simulink model "NLPID"  (Simulink 7.3)
settings: Solver=ode5  StartTime=0.0  StopTime=inf  FixedStep=0.1  RelTol=1e-3
undefined symbols (not defined in the file): eta1_0_real, v1_0_real, velocitySatValues1
libraries: simulink x35, dspmtrx3 x15, simulink_extras x13, dspindex x5, marine_gnc x4, dspinverses x2
(part 4 of 4)

== system NLPID/Control Systems/Nonlinear PID/Thruster allocation/f_act to u_act/f_4 to u_4 ==
  note: If < 0: control input is 1
      | if = 0 control input is 2
      | if > 0: control input is 3
  note: Check if the input value is less, equal or greater then zero
  note: The mapping is divided into 3 parts:
      | Negative, zero and positive
  f_4 : Inport
  Dead Zone : DeadZone  LowerValue=-0.001  UpperValue=0.001  SaturateOnIntegerOverflow=on
  Gain : Gain  Gain=2  ParameterDataType=fixdt(1, 16)  ParameterScaling=2^0  OutDataType=fixdt(1, 16)  OutScaling=2^0
  Gain1 : Gain  Gain=3  ParameterDataType=fixdt(1, 16)  ParameterScaling=2^0  OutDataType=fixdt(1, 16)  OutScaling=2^0
  If < 0 : simulink/Logic and Bit Operations/Compare To Constant  SystemSampleTime=-1  relop=<  const=0  LogicOutDataTypeMode=uint8
  If > 0 : simulink/Logic and Bit Operations/Compare To Constant  SystemSampleTime=-1  relop=>  const=0  LogicOutDataTypeMode=uint8
  Multiport Switch : MultiPortSwitch  OutDataType=fixdt(1, 16)  OutScaling=2^0
  Sum : Sum  Inputs=+++  OutDataType=fixdt(1, 16)  OutScaling=2^0
  f_4 < 0 : Lookup  InputValues=|  Table=|  LookUpMeth=Interpolation-Use End Values  OutDataType=fixdt(1, 16)  OutScaling=2^0
      InputValues=|
      | [-1.249
      | -1.225
      | -1.094
      | -0.896
      | -0.696
      | -0.502
      | -0.314
      | -0.169
      | -0.042
      | 0.000]
      Table=|
      | [-0.9000
      |    -0.8000
      |    -0.7000
      |    -0.6000
      |    -0.5000
      |    -0.4000
      |    -0.3000
      |    -0.2000
      |    -0.1000
      |    -0.0674]
  f_4 = 0 : Constant  Value=0  OutDataType=fixdt(1, 16)  OutScaling=2^0
  f_4 > 0 : Lookup  InputValues=|  Table=|  LookUpMeth=Interpolation-Use End Values  OutDataType=fixdt(1, 16)  OutScaling=2^0
      InputValues=|
      | [0.000
      | 0.063
      | 0.107
      | 0.274
      | 0.441
      | 0.599
      | 0.731]
      Table=|
      | [0.3588
      |     0.5000
      |     0.6000
      |     0.7000
      |     0.8000
      |     0.9000
      |     1.0000]
  if == 0 : simulink/Logic and Bit Operations/Compare To Zero  SystemSampleTime=-1  relop===  LogicOutDataTypeMode=uint8
  u_4 : Outport
  wires:
  f_4 > 0/1 -> Multiport Switch/4
  f_4 = 0/1 -> Multiport Switch/3
  f_4 < 0/1 -> Multiport Switch/2
  f_4/1 -> f_4 > 0/1, f_4 < 0/1, Dead Zone/1
  If < 0/1 -> Sum/1
  if == 0/1 -> Gain/1
  If > 0/1 -> Gain1/1
  Sum/1 -> Multiport Switch/1
  Gain/1 -> Sum/2
  Gain1/1 -> Sum/3
  Multiport Switch/1 -> u_4/1
  Dead Zone/1 -> If > 0/1, if == 0/1, If < 0/1

== system NLPID/Control Systems/Nonlinear PID/Thruster allocation/f_act to u_act/f_5 to u_5 ==
  note: The mapping is divided into 3 parts:
      | Negative, zero and positive
  note: Check if the input value is less, equal or greater then zero
  note: If < 0: control input is 1
      | if = 0 control input is 2
      | if > 0: control input is 3
  f_5 : Inport
  Dead Zone : DeadZone  LowerValue=-0.001  UpperValue=0.001  SaturateOnIntegerOverflow=on
  Gain : Gain  Gain=2  ParameterDataType=fixdt(1, 16)  ParameterScaling=2^0  OutDataType=fixdt(1, 16)  OutScaling=2^0
  Gain1 : Gain  Gain=3  ParameterDataType=fixdt(1, 16)  ParameterScaling=2^0  OutDataType=fixdt(1, 16)  OutScaling=2^0
  If < 0 : simulink/Logic and Bit Operations/Compare To Constant  SystemSampleTime=-1  relop=<  const=0  LogicOutDataTypeMode=uint8
  If > 0 : simulink/Logic and Bit Operations/Compare To Constant  SystemSampleTime=-1  relop=>  const=0  LogicOutDataTypeMode=uint8
  Multiport Switch : MultiPortSwitch  OutDataType=fixdt(1, 16)  OutScaling=2^0
  Sum : Sum  Inputs=+++  OutDataType=fixdt(1, 16)  OutScaling=2^0
  f_5 < 0 : Lookup  InputValues=|  Table=|  LookUpMeth=Interpolation-Use End Values  OutDataType=fixdt(1, 16)  OutScaling=2^0
      InputValues=|
      | [-1.2630
      |    -1.0309
      |    -0.3808]
      Table=|
      | [-0.3000
      |    -0.2000
      |    -0.1000]
  f_5 = 0 : Constant  Value=0  OutDataType=fixdt(1, 16)  OutScaling=2^0
  f_5 > 0 : Lookup  InputValues=|  Table=|  LookUpMeth=Interpolation-Use End Values  OutDataType=fixdt(1, 16)  OutScaling=2^0
      InputValues=|
      | [0.3480
      |     0.8290
      |     1.0930]
      Table=|
      | [0.1000
      |     0.2000
      |     0.3000]
  if == 0 : simulink/Logic and Bit Operations/Compare To Zero  SystemSampleTime=-1  relop===  LogicOutDataTypeMode=uint8
  u_5 : Outport
  wires:
  Multiport Switch/1 -> u_5/1
  Gain1/1 -> Sum/3
  Gain/1 -> Sum/2
  Sum/1 -> Multiport Switch/1
  If > 0/1 -> Gain1/1
  if == 0/1 -> Gain/1
  If < 0/1 -> Sum/1
  f_5/1 -> f_5 < 0/1, f_5 > 0/1, Dead Zone/1
  f_5 < 0/1 -> Multiport Switch/2
  f_5 = 0/1 -> Multiport Switch/3
  f_5 > 0/1 -> Multiport Switch/4
  Dead Zone/1 -> If < 0/1, if == 0/1, If > 0/1

== system NLPID/Control Systems/Nonlinear PID/Thruster allocation/tau to f_act/T_e ==
  -l_x1 : Gain  Gain=-1
  -l_x2 : Gain  Gain=-1
  -l_y2 : Gain  Gain=-1
  3x5 : Reshape  OutputDimensionality=Customize  OutputDimensions=[3,5]
  Mux : Mux  Inputs=15
  T_e{11,13,22,24..25} (5 alike) : Constant
  T_e{12,14..15,21,23} (5 alike) : Constant  Value=0
  l_x1 : Constant  Value=0.45
  l_x2 : Constant  Value=0.45
  l_x3 : Constant  Value=0.385
  l_y1 : Constant  Value=0.055
  l_y2 : Constant  Value=0.055
  T_e : Outport
  wires:
  l_x3/1 -> Mux/15
  T_e25/1 -> Mux/14
  T_e15/1 -> Mux/13
  -l_x2/1 -> Mux/12
  -l_y2/1 -> Mux/9
  -l_x1/1 -> Mux/6
  l_x2/1 -> -l_x2/1
  T_e24/1 -> Mux/11
  T_e14/1 -> Mux/10
  l_y2/1 -> -l_y2/1
  T_e23/1 -> Mux/8
  T_e13/1 -> Mux/7
  l_x1/1 -> -l_x1/1
  T_e22/1 -> Mux/5
  T_e12/1 -> Mux/4
  l_y1/1 -> Mux/3
  T_e21/1 -> Mux/2
  T_e11/1 -> Mux/1
  3x5/1 -> T_e/1
  Mux/1 -> 3x5/1

== system NLPID/Control Systems/PS3 u input control/Subsystem/f_act to tau/T_e ==
  -l_x1 : Gain  Gain=-1
  -l_x2 : Gain  Gain=-1
  -l_y2 : Gain  Gain=-1
  3x5 : Reshape  OutputDimensionality=Customize  OutputDimensions=[3,5]
  Mux : Mux  Inputs=15
  T_e{11,13,22,24..25} (5 alike) : Constant
  T_e{12,14..15,21,23} (5 alike) : Constant  Value=0
  l_x1 : Constant  Value=0.45
  l_x2 : Constant  Value=0.45
  l_x3 : Constant  Value=0.385
  l_y1 : Constant  Value=0.055
  l_y2 : Constant  Value=0.055
  T_e : Outport
  wires:
  Mux/1 -> 3x5/1
  3x5/1 -> T_e/1
  T_e11/1 -> Mux/1
  T_e21/1 -> Mux/2
  l_y1/1 -> Mux/3
  T_e12/1 -> Mux/4
  T_e22/1 -> Mux/5
  l_x1/1 -> -l_x1/1
  T_e13/1 -> Mux/7
  T_e23/1 -> Mux/8
  l_y2/1 -> -l_y2/1
  T_e14/1 -> Mux/10
  T_e24/1 -> Mux/11
  l_x2/1 -> -l_x2/1
  -l_x1/1 -> Mux/6
  -l_y2/1 -> Mux/9
  -l_x2/1 -> Mux/12
  T_e15/1 -> Mux/13
  T_e25/1 -> Mux/14
  l_x3/1 -> Mux/15

== system NLPID/Guidance Systems/Path-following/Heading/psi_d eq/rad to pi2pi ==
  note: r
  note: x
  x (rad) : Inport  OutDataType=sfix(16)  OutScaling=2^0
  Constant : Constant  Value=2*180  OutDataType=sfix(16)  OutScaling=2^0
  Degrees to Radians : simulink_extras/Transformations/Degrees to Radians  SystemSampleTime=-1
  Gain : Gain  Gain=180  ParameterDataType=sfix(16)  ParameterScaling=2^0  OutDataType=sfix(16)  OutScaling=2^0  SaturateOnIntegerOverflow=on  OutDataTypeStr=Inherit: Same as input  ParamDataTypeStr=Inherit: Same as input
  Math Function : Math  Operator=rem  OutDataType=sfix(16)  OutScaling=2^0  SaturateOnIntegerOverflow=on
  Radians to Degrees : simulink_extras/Transformations/Radians to Degrees  SystemSampleTime=-1
  Saturation : Saturate  UpperLimit=1e10  LowerLimit=-1e10
  Sign : Signum
  Sum : Sum  Inputs=|+-  OutDataType=sfix(16)  OutScaling=2^0  SaturateOnIntegerOverflow=on
  Sum1 : Sum  Inputs=|++  OutDataType=sfix(16)  OutScaling=2^0  SaturateOnIntegerOverflow=on
  -pi to pi : Outport  OutDataType=sfix(16)  OutScaling=2^0
  wires:
  Radians to Degrees/1 -> Saturation/1
  Degrees to Radians/1 -> -pi to pi/1
  Sum/1 -> Degrees to Radians/1
  Math Function/1 -> Sum/1
  Constant/1 -> Math Function/2
  Sum1/1 -> Math Function/1
  Gain/1 -> Sum1/2, Sum/2
  Sign/1 -> Gain/1
  x (rad)/1 -> Radians to Degrees/1
  Saturation/1 -> Sign/1, Sum1/1

== system NLPID/Guidance Systems/Path-following/Line-Of-Sight/Dynamic LOS assigment for qdot/f_q eq ==
  psi_los : Inport
  u_d : Inport  Port=2
  Mux : Mux  Inputs=2
  Product : Product  Multiplication=Matrix(*)  OutDataType=fixdt(1, 16)  OutScaling=2^0  RndMeth=Zero
  f_qx : Trigonometry  Operator=cos
  f_qy : Trigonometry
  f_q : Outport
  wires:
  psi_los/1 -> f_qx/1, f_qy/1
  f_qx/1 -> Mux/1
  f_qy/1 -> Mux/2
  Mux/1 -> Product/1
  u_d/1 -> Product/2
  Product/1 -> f_q/1

== system NLPID/Guidance Systems/Path-following/Line-Of-Sight/Dynamic LOS assigment for qdot/f_q^q eq ==
  psi_los : Inport
  u_d : Inport  Port=2
  psi_los^q : Inport  Port=3
  Gain : Gain  Gain=-1  ParameterDataType=fixdt(1, 16)  ParameterScaling=2^0  OutDataType=fixdt(1, 16)  OutScaling=2^0
  Matrix Concatenate : Concatenate  Mode=Multidimensional array
  Product : Product  OutDataType=fixdt(1, 16)  OutScaling=2^0  RndMeth=Zero
  Product1 : Product  Multiplication=Matrix(*)  OutDataType=fixdt(1, 16)  OutScaling=2^0  RndMeth=Zero
  Product2 : Product  Multiplication=Matrix(*)  OutDataType=fixdt(1, 16)  OutScaling=2^0  RndMeth=Zero
  Trigonometric Function : Trigonometry  Operator=cos
  Trigonometric Function1 : Trigonometry
  "f_q^q " : Outport
  wires:
  psi_los/1 -> Trigonometric Function1/1, Trigonometric Function/1
  u_d/1 -> Product/2
  Product/1 -> "f_q^q "/1
  Trigonometric Function1/1 -> Gain/1
  Gain/1 -> Product1/1
  psi_los^q/1 -> Product1/2, Product2/2
  Trigonometric Function/1 -> Product2/1
  Product1/1 -> Matrix Concatenate/1
  Product2/1 -> Matrix Concatenate/2
  Matrix Concatenate/1 -> Product/1

== system NLPID/Guidance Systems/Path-following/Line-Of-Sight/Dynamic LOS assigment for qdot/f_q^s eq ==
  psi_los : Inport
  u_d : Inport  Port=2
  psi_los^s : Inport  Port=3
  Gain : Gain  Gain=-1  ParameterDataType=fixdt(1, 16)  ParameterScaling=2^0  OutDataType=fixdt(1, 16)  OutScaling=2^0
  Mux : Mux  Inputs=2
  Product : Product  Multiplication=Matrix(*)  OutDataType=fixdt(1, 16)  OutScaling=2^0  RndMeth=Zero
  Product1 : Product  OutDataType=fixdt(1, 16)  OutScaling=2^0  RndMeth=Zero
  Product2 : Product  OutDataType=fixdt(1, 16)  OutScaling=2^0  RndMeth=Zero
  Trigonometric Function : Trigonometry  Operator=cos
  Trigonometric Function1 : Trigonometry
  f_q^s : Outport
  wires:
  psi_los/1 -> Trigonometric Function1/1, Trigonometric Function/1
  u_d/1 -> Product/2
  Product/1 -> f_q^s/1
  Trigonometric Function1/1 -> Gain/1
  Gain/1 -> Product1/1
  psi_los^s/1 -> Product1/2, Product2/2
  Trigonometric Function/1 -> Product2/1
  Product1/1 -> Mux/1
  Product2/1 -> Mux/2
  Mux/1 -> Product/1

== system NLPID/Guidance Systems/Path-following/Line-Of-Sight/Dynamic LOS assigment for qdot/f_q^t eq ==
  psi_los : Inport
  u_d^t : Inport  Port=2
  Mux : Mux  Inputs=2
  Product : Product  OutDataType=fixdt(1, 16)  OutScaling=2^0  RndMeth=Zero
  Trigonometric Function : Trigonometry  Operator=cos
  Trigonometric Function1 : Trigonometry
  f_q^t : Outport
  wires:
  psi_los/1 -> Trigonometric Function/1, Trigonometric Function1/1
  Trigonometric Function/1 -> Mux/1
  Trigonometric Function1/1 -> Mux/2
  Mux/1 -> Product/1
  u_d^t/1 -> Product/2
  Product/1 -> f_q^t/1

== system NLPID/Guidance Systems/Path-following/Line-Of-Sight/Dynamic assigment for sdot/f_s eq ==
  Delta : Inport
  epsilon_n : Inport  Port=2
  v_s : Inport  Port=3
  omega_s : Inport  Port=4
  Add : Sum  OutDataType=fixdt(1, 16)  OutScaling=2^-10
  Delta^2 : Math  Operator=square  OutDataType=fixdt(1, 16)  OutScaling=2^0  SaturateOnIntegerOverflow=on
  Divide : Product  Inputs=*/  OutDataType=fixdt(1, 16)  OutScaling=2^-10
  Product : Product  OutDataType=fixdt(1, 16)  OutScaling=2^0  RndMeth=Zero
  Scope{,1..3} (4 alike) : Scope
      Scope settings: SaveName=ScopeData12
      Scope1 settings: SaveName=ScopeData13
      Scope2 settings: SaveName=ScopeData14
      Scope3 settings: SaveName=ScopeData15
  Subtract : Sum  Inputs=+-  OutDataType=fixdt(1, 16)  OutScaling=2^-10
  epsilon_n^2 : Math  Operator=square  OutDataType=fixdt(1, 16)  OutScaling=2^0  SaturateOnIntegerOverflow=on
  sqrt : Math  Operator=sqrt  OutDataType=fixdt(1, 16)  OutScaling=2^0  SaturateOnIntegerOverflow=on
  f_s : Outport
  wires:
  epsilon_n/1 -> epsilon_n^2/1
  Delta/1 -> Delta^2/1, Divide/1, Scope2/1
  Add/1 -> sqrt/1
  sqrt/1 -> Divide/2, Scope/1
  v_s/1 -> Product/2
  Subtract/1 -> f_s/1, Scope3/1
  epsilon_n^2/1 -> Add/1
  Delta^2/1 -> Add/2
  omega_s/1 -> Subtract/2
  Product/1 -> Subtract/1
  Divide/1 -> Product/1, Scope1/1

== system NLPID/Guidance Systems/Path-following/Line-Of-Sight/Dynamic assigment for sdot/f_s^q eq ==
  Delta : Inport
  epsilon_n : Inport  Port=2
  v_s : Inport  Port=3
  omega_s^q : Inport  Port=4
  epsilon_n^q : Inport  Port=5
  3/2 : Constant  Value=3/2  OutDataType=fixdt(1, 16)  OutScaling=2^0
  Add : Sum  OutDataType=fixdt(1, 16)  OutScaling=2^-10
  Delta^2 : Math  Operator=square  OutDataType=fixdt(1, 16)  OutScaling=2^0  SaturateOnIntegerOverflow=on
  Divide : Product  Inputs=*/  OutDataType=fixdt(1, 16)  OutScaling=2^-10
  Product : Product  Inputs=3  OutDataType=fixdt(1, 16)  OutScaling=2^0  RndMeth=Zero
  Product1 : Product  OutDataType=fixdt(1, 16)  OutScaling=2^0  RndMeth=Zero
  Sum : Sum  Inputs=--  OutDataType=fixdt(1, 16)  OutScaling=2^-10
  ^3/2 : Math  Operator=pow  OutDataType=fixdt(1, 16)  OutScaling=2^0  SaturateOnIntegerOverflow=on
  epsilon_n^2 : Math  Operator=square  OutDataType=fixdt(1, 16)  OutScaling=2^0  SaturateOnIntegerOverflow=on
  f_s^q : Outport
  wires:
  epsilon_n/1 -> epsilon_n^2/1, Product1/1
  Delta/1 -> Delta^2/1, Product/1
  Add/1 -> ^3/2/1
  ^3/2/1 -> Divide/2
  Product/1 -> Sum/1
  omega_s^q/1 -> Sum/2
  Sum/1 -> f_s^q/1
  epsilon_n^2/1 -> Add/1
  Delta^2/1 -> Add/2
  v_s/1 -> Product/3
  epsilon_n^q/1 -> Product1/2
  Product1/1 -> Divide/1
  3/2/1 -> ^3/2/2
  Divide/1 -> Product/2

== system NLPID/Guidance Systems/Path-following/Line-Of-Sight/Dynamic assigment for sdot/f_s^s eq ==
  Delta : Inport
  epsilon_n : Inport  Port=2
  v_s : Inport  Port=3
  omega_s^s : Inport  Port=4
  epsilon_n^s : Inport  Port=5
  v_s^s : Inport  Port=6
  3/2 : Constant  Value=3/2  OutDataType=fixdt(1, 16)  OutScaling=2^0
  Add : Sum  OutDataType=fixdt(1, 16)  OutScaling=2^-10
  Delta^2 : Math  Operator=square  OutDataType=fixdt(1, 16)  OutScaling=2^0  SaturateOnIntegerOverflow=on
  Divide : Product  Inputs=*/  OutDataType=fixdt(1, 16)  OutScaling=2^-10
  Divide1 : Product  Inputs=*/  OutDataType=fixdt(1, 16)  OutScaling=2^-10
  Math Function : Math  Operator=sqrt  OutDataType=fixdt(1, 16)  OutScaling=2^0  SaturateOnIntegerOverflow=on
  Product1 : Product  OutDataType=fixdt(1, 16)  OutScaling=2^0  RndMeth=Zero
  Product2 : Product  OutDataType=fixdt(1, 16)  OutScaling=2^0  RndMeth=Zero
  Product3 : Product  Inputs=3  OutDataType=fixdt(1, 16)  OutScaling=2^0  RndMeth=Zero
  Sum : Sum  Inputs=+--  OutDataType=fixdt(1, 16)  OutScaling=2^-10
  ^3/2 : Math  Operator=pow  OutDataType=fixdt(1, 16)  OutScaling=2^0  SaturateOnIntegerOverflow=on
  epsilon_n^2 : Math  Operator=square  OutDataType=fixdt(1, 16)  OutScaling=2^0  SaturateOnIntegerOverflow=on
  f_s^s : Outport
  wires:
  Delta/1 -> Product1/1, Delta^2/1, Product3/1
  Add/1 -> Math Function/1, ^3/2/1
  Sum/1 -> f_s^s/1
  epsilon_n^2/1 -> Add/1
  Delta^2/1 -> Add/2
  omega_s^s/1 -> Sum/3
  v_s^s/1 -> Divide/1
  epsilon_n/1 -> epsilon_n^2/1, Product2/1
  3/2/1 -> ^3/2/2
  Math Function/1 -> Divide/2
  Divide/1 -> Product1/2
  Product1/1 -> Sum/1
  v_s/1 -> Product3/3
  Divide1/1 -> Product3/2
  epsilon_n^s/1 -> Product2/2
  Product2/1 -> Divide1/1
  ^3/2/1 -> Divide1/2
  Product3/1 -> Sum/2

== system NLPID/Guidance Systems/Path-following/Line-Of-Sight/Dynamic assigment for sdot/f_t eq ==
  Delta : Inport
  epsilon_n : Inport  Port=2
  v_s^t : Inport  Port=3
  Add : Sum  OutDataType=fixdt(1, 16)  OutScaling=2^-10
  Delta^2 : Math  Operator=square  OutDataType=fixdt(1, 16)  OutScaling=2^0  SaturateOnIntegerOverflow=on
  Divide : Product  Inputs=*/  OutDataType=fixdt(1, 16)  OutScaling=2^-10
  Product : Product  OutDataType=fixdt(1, 16)  OutScaling=2^0  RndMeth=Zero
  epsilon_n^2 : Math  Operator=square  OutDataType=fixdt(1, 16)  OutScaling=2^0  SaturateOnIntegerOverflow=on
  sqrt : Math  Operator=sqrt  OutDataType=fixdt(1, 16)  OutScaling=2^0  SaturateOnIntegerOverflow=on
  f_t : Outport
  wires:
  epsilon_n/1 -> epsilon_n^2/1
  Delta/1 -> Delta^2/1, Divide/1
  Add/1 -> sqrt/1
  sqrt/1 -> Divide/2
  Divide/1 -> Product/1
  v_s^t/1 -> Product/2
  Product/1 -> f_t/1
  epsilon_n^2/1 -> Add/1
  Delta^2/1 -> Add/2

== system NLPID/Guidance Systems/Path-following/Line-Of-Sight/Gradient update law for sdot/omega_s eq ==
  p_d^s : Inport
  q - p_d : Inport  Port=2
  my : Inport  Port=3
  |p_d^s| : Inport  Port=4
  Divide : Product  Inputs=*/  OutDataType=fixdt(1, 16)  OutScaling=2^-10
  Gain : Gain  Gain=-1  ParameterDataType=fixdt(1, 16)  ParameterScaling=2^0  OutDataType=fixdt(1, 16)  OutScaling=2^0
  Product : Product  Inputs=3  Multiplication=Matrix(*)  OutDataType=fixdt(1, 16)  OutScaling=2^0  RndMeth=Zero
  Transpose : dspmtrx3/Transpose  SystemSampleTime=-1  Hermitian=off  overflowFlag=off
  omega_s : Outport
  wires:
  my/1 -> Product/1
  p_d^s/1 -> Transpose/1
  Transpose/1 -> Divide/1
  Divide/1 -> Product/2
  Product/1 -> Gain/1
  Gain/1 -> omega_s/1
  |p_d^s|/1 -> Divide/2
  q - p_d/1 -> Product/3

== system NLPID/Guidance Systems/Path-following/Line-Of-Sight/Gradient update law for sdot/omega_s^q eq ==
  p_d^s : Inport
  my : Inport  Port=2
  |p_d^s| : Inport  Port=3
  Divide : Product  Inputs=*/  OutDataType=fixdt(1, 16)  OutScaling=2^-10
  Gain : Gain  Gain=-1  ParameterDataType=fixdt(1, 16)  ParameterScaling=2^0  OutDataType=fixdt(1, 16)  OutScaling=2^0
  Product : Product  Multiplication=Matrix(*)  OutDataType=fixdt(1, 16)  OutScaling=2^0  RndMeth=Zero
  Transpose : dspmtrx3/Transpose  SystemSampleTime=-1  Hermitian=off  overflowFlag=off
  omega_s^q : Outport
  wires:
  my/1 -> Product/1
  p_d^s/1 -> Transpose/1
  Transpose/1 -> Divide/1
  Divide/1 -> Product/2
  Product/1 -> Gain/1
  Gain/1 -> omega_s^q/1
  |p_d^s|/1 -> Divide/2

== system NLPID/Guidance Systems/Path-following/Line-Of-Sight/Gradient update law for sdot/omega_s^s eq ==
  p_d^s : Inport
  q - p_d : Inport  Port=2
  my : Inport  Port=3
  |p_d^s| : Inport  Port=4
  p_d^s^2 : Inport  Port=5
  Constant : Constant  Value=3  OutDataType=fixdt(1, 16)  OutScaling=2^0
  Divide1 : Product  Inputs=*/  OutDataType=fixdt(1, 16)  OutScaling=2^-10
  Divide2 : Product  Inputs=*/  OutDataType=fixdt(1, 16)  OutScaling=2^-10
  Math Function : Math  Operator=pow  OutDataType=fixdt(1, 16)  OutScaling=2^0  SaturateOnIntegerOverflow=on
  Product : Product  Inputs=3  Multiplication=Matrix(*)  OutDataType=fixdt(1, 16)  OutScaling=2^0  RndMeth=Zero
  Product1 : Product  OutDataType=fixdt(1, 16)  OutScaling=2^0  RndMeth=Zero
  Product2 : Product  Inputs=3  Multiplication=Matrix(*)  OutDataType=fixdt(1, 16)  OutScaling=2^0  RndMeth=Zero
  Subtract : Sum  Inputs=+-  OutDataType=fixdt(1, 16)  OutScaling=2^-10
  Subtract1 : Sum  Inputs=+-  OutDataType=fixdt(1, 16)  OutScaling=2^-10
  Transpose1 : dspmtrx3/Transpose  SystemSampleTime=-1  Hermitian=off  overflowFlag=off
  Transpose2 : dspmtrx3/Transpose  SystemSampleTime=-1  Hermitian=off  overflowFlag=off
  omega_s^s : Outport
  wires:
  Product/1 -> Subtract/2
  my/1 -> Product1/1, Product/1
  |p_d^s|/1 -> Product1/2, Math Function/1, Divide2/2
  Product1/1 -> Subtract/1
  Subtract/1 -> omega_s^s/1
  p_d^s^2/1 -> Transpose2/1
  Transpose1/1 -> Product2/3
  p_d^s/1 -> Transpose1/1, Product2/2
  Product2/1 -> Divide1/1
  Constant/1 -> Math Function/2
  Math Function/1 -> Divide1/2
  Divide1/1 -> Subtract1/2
  Subtract1/1 -> Product/2
  q - p_d/1 -> Product/3
  Transpose2/1 -> Divide2/1, Product2/1
  Divide2/1 -> Subtract1/1

== system NLPID/Guidance Systems/Path-following/Line-Of-Sight/LOS heading/psi_los eq ==
  psi_d : Inport
  epsilon_n : Inport  Port=2
  Delta : Inport  Port=3
  Subtract : Sum  Inputs=+-  OutDataType=fixdt(1, 16)  OutScaling=2^-10
  Trigonometric Function : Trigonometry  Operator=atan2
  rad to pi2pi1 : Subsystem  AncestorBlock=marine_gnc/Utilities/Math Operations/deg to 180//180
      mask Type: rad to pi/pi
      mask Description: Converts an angle in rad to +- pi
      mask Display: disp('[0 2pi] to [-pi pi]')
  rad to pi2pi2 : Subsystem  AncestorBlock=marine_gnc/Utilities/Math Operations/deg to 180//180
      mask Type: rad to pi/pi
      mask Description: Converts an angle in rad to +- pi
      mask Display: disp('[0 2pi] to [-pi pi]')
  rad to pi2pi3 : Subsystem  AncestorBlock=marine_gnc/Utilities/Math Operations/deg to 180//180
      mask Type: rad to pi/pi
      mask Description: Converts an angle in rad to +- pi
      mask Display: disp('[0 2pi] to [-pi pi]')
  psi_los : Outport
  wires:
  psi_d/1 -> rad to pi2pi1/1(x (rad))
  Trigonometric Function/1 -> rad to pi2pi2/1(x (rad))
  Delta/1 -> Trigonometric Function/2
  epsilon_n/1 -> Trigonometric Function/1
  Subtract/1 -> rad to pi2pi3/1(x (rad))
  rad to pi2pi2/1(-pi to pi) -> Subtract/2
  rad to pi2pi3/1(-pi to pi) -> psi_los/1
  rad to pi2pi1/1(-pi to pi) -> Subtract/1

== system NLPID/Guidance Systems/Path-following/Line-Of-Sight/LOS heading/psi_los^q eq ==
  epsilon_n : Inport
  Delta : Inport  Port=2
  epsilon_n^q : Inport  Port=3
  -1 : Gain  Gain=-1  ParameterDataType=fixdt(1, 16)  ParameterScaling=2^0  OutDataType=fixdt(1, 16)  OutScaling=2^0
  Add : Sum  Inputs=|++  OutDataType=fixdt(1, 16)  OutScaling=2^-10
  Delta^2 : Math  Operator=square  OutDataType=fixdt(1, 16)  OutScaling=2^0  SaturateOnIntegerOverflow=on
  Divide : Product  Inputs=*/  OutDataType=fixdt(1, 16)  OutScaling=2^-10
  Product : Product  OutDataType=fixdt(1, 16)  OutScaling=2^0  RndMeth=Zero
  epsilon_n^2 : Math  Operator=square  OutDataType=fixdt(1, 16)  OutScaling=2^0  SaturateOnIntegerOverflow=on
  psi_los^q : Outport
  wires:
  epsilon_n/1 -> epsilon_n^2/1
  epsilon_n^2/1 -> Add/2
  Add/1 -> Divide/2
  Divide/1 -> Product/1
  epsilon_n^q/1 -> Product/2
  Product/1 -> -1/1
  -1/1 -> psi_los^q/1
  Delta^2/1 -> Add/1
  Delta/1 -> Divide/1, Delta^2/1

== system NLPID/Guidance Systems/Path-following/Line-Of-Sight/LOS heading/psi_los^q^2 eq ==
  epsilon_n : Inport
  Delta : Inport  Port=2
  epsilon_n^q : Inport  Port=3
  epsilon_n^q^2 : Inport  Port=4
  ( )^2 : Math  Operator=square  OutDataType=fixdt(1, 16)  OutScaling=2^0  SaturateOnIntegerOverflow=on
  2 : Gain  Gain=2  ParameterDataType=fixdt(1, 16)  ParameterScaling=2^0  OutDataType=fixdt(1, 16)  OutScaling=2^0
  Add : Sum  Inputs=|++  OutDataType=fixdt(1, 16)  OutScaling=2^-10
  Delta^2 : Math  Operator=square  OutDataType=fixdt(1, 16)  OutScaling=2^0  SaturateOnIntegerOverflow=on
  Divide : Product  Inputs=*/  OutDataType=fixdt(1, 16)  OutScaling=2^-10
  Divide1 : Product  Inputs=*/  OutDataType=fixdt(1, 16)  OutScaling=2^-10
  Math Function : Math  Operator=transpose  OutDataType=fixdt(1, 16)  OutScaling=2^0  SaturateOnIntegerOverflow=on
  Product1 : Product  OutDataType=fixdt(1, 16)  OutScaling=2^0  RndMeth=Zero
  Product2 : Product  OutDataType=fixdt(1, 16)  OutScaling=2^0  RndMeth=Zero
  Product3 : Product  Multiplication=Matrix(*)  OutDataType=fixdt(1, 16)  OutScaling=2^0  RndMeth=Zero
  Product4 : Product  OutDataType=fixdt(1, 16)  OutScaling=2^0  RndMeth=Zero
  Subtract : Sum  Inputs=|+-  OutDataType=fixdt(1, 16)  OutScaling=2^-10
  epsilon_n^2 : Math  Operator=square  OutDataType=fixdt(1, 16)  OutScaling=2^0  SaturateOnIntegerOverflow=on
  psi_los^q^2 : Outport
  wires:
  Subtract/1 -> psi_los^q^2/1
  Divide/1 -> Subtract/1
  2/1 -> Divide/1
  Delta/1 -> Product2/1, Product1/1, Delta^2/1
  epsilon_n^q/1 -> Math Function/1, Product3/2
  Delta^2/1 -> Add/1
  Add/1 -> ( )^2/1, Divide1/2
  epsilon_n^2/1 -> Add/2
  ( )^2/1 -> Divide/2
  epsilon_n^q^2/1 -> Product1/2
  Product1/1 -> Divide1/1
  Divide1/1 -> Subtract/2
  epsilon_n/1 -> epsilon_n^2/1, Product2/2
  Math Function/1 -> Product3/1
  Product3/1 -> Product4/2
  Product2/1 -> Product4/1
  Product4/1 -> 2/1

== system NLPID/Guidance Systems/Path-following/Line-Of-Sight/LOS heading/psi_los^qs = psi_los^sq ==
  epsilon_n : Inport
  Delta : Inport  Port=2
  epsilon_n^s : Inport  Port=3
  epsilon_n^q : Inport  Port=4
  epsilon_n^qs : Inport  Port=5
  ( )^2 : Math  Operator=square  OutDataType=fixdt(1, 16)  OutScaling=2^0  SaturateOnIntegerOverflow=on
  2 : Gain  Gain=2  ParameterDataType=fixdt(1, 16)  ParameterScaling=2^0  OutDataType=fixdt(1, 16)  OutScaling=2^0
  Add : Sum  Inputs=|++  OutDataType=fixdt(1, 16)  OutScaling=2^-10
  Delta^2 : Math  Operator=square  OutDataType=fixdt(1, 16)  OutScaling=2^0  SaturateOnIntegerOverflow=on
  Divide : Product  Inputs=*/  OutDataType=fixdt(1, 16)  OutScaling=2^-10
  Divide1 : Product  Inputs=*/  OutDataType=fixdt(1, 16)  OutScaling=2^-10
  Product : Product  Inputs=4  Multiplication=Matrix(*)  OutDataType=fixdt(1, 16)  OutScaling=2^0  RndMeth=Zero
  Product1 : Product  Multiplication=Matrix(*)  OutDataType=fixdt(1, 16)  OutScaling=2^0  RndMeth=Zero
  Subtract : Sum  Inputs=|+-  OutDataType=fixdt(1, 16)  OutScaling=2^-10
  epsilon_n^2 : Math  Operator=square  OutDataType=fixdt(1, 16)  OutScaling=2^0  SaturateOnIntegerOverflow=on
  psi_los^qs : Outport
  wires:
  Subtract/1 -> psi_los^qs/1
  Divide/1 -> Subtract/1
  Delta/1 -> Product/1, Delta^2/1, Product1/1
  epsilon_n/1 -> Product/2, epsilon_n^2/1
  epsilon_n^s/1 -> Product/3
  epsilon_n^q/1 -> Product/4
  Product/1 -> 2/1
  epsilon_n^2/1 -> Add/2
  Add/1 -> ( )^2/1, Divide1/2
  Delta^2/1 -> Add/1
  ( )^2/1 -> Divide/2
  epsilon_n^qs/1 -> Product1/2
  Product1/1 -> Divide1/1
  Divide1/1 -> Subtract/2
  2/1 -> Divide/1

== system NLPID/Guidance Systems/Path-following/Line-Of-Sight/LOS heading/psi_los^s eq ==
  epsilon_n : Inport
  Delta : Inport  Port=2
  psi_d^s : Inport  Port=3
  epsilon_n^s : Inport  Port=4
  Add : Sum  Inputs=|++  OutDataType=fixdt(1, 16)  OutScaling=2^-10
  Delta^2 : Math  Operator=square  OutDataType=fixdt(1, 16)  OutScaling=2^0  SaturateOnIntegerOverflow=on
  Divide : Product  Inputs=*/  OutDataType=fixdt(1, 16)  OutScaling=2^-10
  Product : Product  OutDataType=fixdt(1, 16)  OutScaling=2^0  RndMeth=Zero
  Subtract : Sum  Inputs=|+-  OutDataType=fixdt(1, 16)  OutScaling=2^-10
  epsilon_n^2 : Math  Operator=square  OutDataType=fixdt(1, 16)  OutScaling=2^0  SaturateOnIntegerOverflow=on
  psi_los^s : Outport
  wires:
  Divide/1 -> Product/1
  epsilon_n^s/1 -> Product/2
  psi_d^s/1 -> Subtract/1
  Product/1 -> Subtract/2
  Subtract/1 -> psi_los^s/1
  epsilon_n/1 -> epsilon_n^2/1
  epsilon_n^2/1 -> Add/2
  Add/1 -> Divide/2
  Delta^2/1 -> Add/1
  Delta/1 -> Delta^2/1, Divide/1

== system NLPID/Guidance Systems/Path-following/Line-Of-Sight/LOS heading/psi_los^s^2 eq ==
  epsilon_n : Inport
  Delta : Inport  Port=2
  epsilon_n^s : Inport  Port=3
  psi_d¨^s^2 : Inport  Port=4
  epsilon_n^s^2 : Inport  Port=5
  ( )^2 : Math  Operator=square  OutDataType=fixdt(1, 16)  OutScaling=2^0  SaturateOnIntegerOverflow=on
  (epsilon_n^s)^2 : Math  Operator=square  OutDataType=fixdt(1, 16)  OutScaling=2^0  SaturateOnIntegerOverflow=on
  2 : Gain  Gain=2  ParameterDataType=fixdt(1, 16)  ParameterScaling=2^0  OutDataType=fixdt(1, 16)  OutScaling=2^0
  Add : Sum  Inputs=|++  OutDataType=fixdt(1, 16)  OutScaling=2^-10
  Delta^2 : Math  Operator=square  OutDataType=fixdt(1, 16)  OutScaling=2^0  SaturateOnIntegerOverflow=on
  Divide : Product  Inputs=*/  OutDataType=fixdt(1, 16)  OutScaling=2^-10
  Divide1 : Product  Inputs=*/  OutDataType=fixdt(1, 16)  OutScaling=2^-10
  Product : Product  Inputs=3  Multiplication=Matrix(*)  OutDataType=fixdt(1, 16)  OutScaling=2^0  RndMeth=Zero
  Product1 : Product  Multiplication=Matrix(*)  OutDataType=fixdt(1, 16)  OutScaling=2^0  RndMeth=Zero
  Sum : Sum  Inputs=++-  OutDataType=fixdt(1, 16)  OutScaling=2^-10
  epsilon_n^2 : Math  Operator=square  OutDataType=fixdt(1, 16)  OutScaling=2^0  SaturateOnIntegerOverflow=on
  psi_los^s^2 : Outport
  wires:
  Sum/1 -> psi_los^s^2/1
  psi_d¨^s^2/1 -> Sum/1
  Divide/1 -> Sum/2
  Delta/1 -> Product/1, Delta^2/1, Product1/1
  epsilon_n/1 -> Product/2, epsilon_n^2/1
  (epsilon_n^s)^2/1 -> Product/3
  Product/1 -> 2/1
  epsilon_n^2/1 -> Add/2
  Add/1 -> ( )^2/1, Divide1/2
  Delta^2/1 -> Add/1
  ( )^2/1 -> Divide/2
  Product1/1 -> Divide1/1
  Divide1/1 -> Sum/3
  2/1 -> Divide/1
  epsilon_n^s/1 -> (epsilon_n^s)^2/1
  epsilon_n^s^2/1 -> Product1/2

== system NLPID/Guidance Systems/Path-following/Line-Of-Sight/Position error signals/R_2 ==
  psi_d : Inport
  Mux : Mux
  R11 : Trigonometry  Operator=cos
  R12 : Gain  Gain=-1  ParameterDataType=fixdt(1, 16)  ParameterScaling=2^0  OutDataType=fixdt(1, 16)  OutScaling=2^0
  R21 : Trigonometry
  R22 : Gain  ParameterDataType=fixdt(1, 16)  ParameterScaling=2^0  OutDataType=fixdt(1, 16)  OutScaling=2^0
  R_2(psi_d) : Reshape  OutputDimensionality=Customize  OutputDimensions=[2,2]
  R_2 : Outport
  wires:
  R_2(psi_d)/1 -> R_2/1
  Mux/1 -> R_2(psi_d)/1
  R21/1 -> R12/1, Mux/2
  psi_d/1 -> R21/1, R11/1
  R11/1 -> Mux/1, R22/1
  R12/1 -> Mux/3
  R22/1 -> Mux/4

== system NLPID/Guidance Systems/Path-following/Line-Of-Sight/Position error signals/S_2 ==
  psi_d^s : Inport
  0 : Constant  Value=0  OutDataType=fixdt(1, 16)  OutScaling=2^0
  Mux : Mux
  S12 : Gain  Gain=-1  ParameterDataType=fixdt(1, 16)  ParameterScaling=2^0  OutDataType=fixdt(1, 16)  OutScaling=2^0
  S_2(psi_d^s) : Reshape  OutputDimensionality=Customize  OutputDimensions=[2,2]
  S_2 : Outport
  wires:
  S_2(psi_d^s)/1 -> S_2/1
  Mux/1 -> S_2(psi_d^s)/1
  psi_d^s/1 -> S12/1, Mux/2
  S12/1 -> Mux/3
  0/1 -> Mux/4, Mux/1

== system NLPID/Guidance Systems/Path-following/Line-Of-Sight/Position error signals/S_2(psi_d^s^2) ==
  psi_d^s^2 : Inport
  0 : Constant  Value=0  OutDataType=fixdt(1, 16)  OutScaling=2^0
  Mux : Mux
  S12 : Gain  Gain=-1  ParameterDataType=fixdt(1, 16)  ParameterScaling=2^0  OutDataType=fixdt(1, 16)  OutScaling=2^0
  S_2(psi_d^s^2) : Reshape  OutputDimensionality=Customize  OutputDimensions=[2,2]
  S_2 : Outport
  wires:
  0/1 -> Mux/1, Mux/4
  S12/1 -> Mux/3
  psi_d^s^2/1 -> Mux/2, S12/1
  Mux/1 -> S_2(psi_d^s^2)/1
  S_2(psi_d^s^2)/1 -> S_2/1

== system NLPID/Guidance Systems/Path-following/Line-Of-Sight/Position error signals/epsilon^qs = epsilon^sq ==
  R_2^T : Inport
  S_2^T : Inport  Port=2
  Product1 : Product  Multiplication=Matrix(*)  OutDataType=fixdt(1, 16)  OutScaling=2^0  RndMeth=Zero
  epsilon^qs : Outport
  wires:
  Product1/1 -> epsilon^qs/1
  S_2^T/1 -> Product1/1
  R_2^T/1 -> Product1/2

== system NLPID/Guidance Systems/Path-following/Line-Of-Sight/Position error signals/epsilon^s eq ==
  q - p_d : Inport
  R_2^T : Inport  Port=2
  S_2^T : Inport  Port=3
  p_d^s : Inport  Port=4
  Product : Product  Inputs=3  Multiplication=Matrix(*)  OutDataType=fixdt(1, 16)  OutScaling=2^0  RndMeth=Zero
  Product1 : Product  Multiplication=Matrix(*)  OutDataType=fixdt(1, 16)  OutScaling=2^0  RndMeth=Zero
  Subtract1 : Sum  Inputs=+-  OutDataType=fixdt(1, 16)  OutScaling=2^-10
  epsilon^s : Outport
  wires:
  S_2^T/1 -> Product/1
  R_2^T/1 -> Product/2, Product1/1
  p_d^s/1 -> Product1/2
  Product/1 -> Subtract1/1
  Product1/1 -> Subtract1/2
  Subtract1/1 -> epsilon^s/1
  q - p_d/1 -> Product/3

== system NLPID/Guidance Systems/Path-following/Line-Of-Sight/Position error signals/epsilon^s^2 eq ==
  q - p_d : Inport
  p_d^s : Inport  Port=2
  R_2^T : Inport  Port=3
  S_2^T : Inport  Port=4
  S_2(psi_d^s^2)^T : Inport  Port=5
  p_d^s^2 : Inport  Port=6
  2 : Gain  Gain=2  ParameterDataType=fixdt(1, 16)  ParameterScaling=2^0  OutDataType=fixdt(1, 16)  OutScaling=2^0
  Add : Sum  OutDataType=fixdt(1, 16)  OutScaling=2^-10
  Gain : Gain  ParameterDataType=fixdt(1, 16)  ParameterScaling=2^0  OutDataType=fixdt(1, 16)  OutScaling=2^0
  Product : Product  Multiplication=Matrix(*)  OutDataType=fixdt(1, 16)  OutScaling=2^0  RndMeth=Zero
  Product1 : Product  Inputs=3  Multiplication=Matrix(*)  OutDataType=fixdt(1, 16)  OutScaling=2^0  RndMeth=Zero
  Product2 : Product  Inputs=3  Multiplication=Matrix(*)  OutDataType=fixdt(1, 16)  OutScaling=2^0  RndMeth=Zero
  Product3 : Product  Multiplication=Matrix(*)  OutDataType=fixdt(1, 16)  OutScaling=2^0  RndMeth=Zero
  Sum : Sum  Inputs=+--  OutDataType=fixdt(1, 16)  OutScaling=2^-10
  epsilon^s^2 : Outport
  wires:
  Sum/1 -> Gain/1
  Product2/1 -> 2/1
  Gain/1 -> epsilon^s^2/1
  S_2(psi_d^s^2)^T/1 -> Add/1
  S_2^T/1 -> Product/1, Product2/1, Product/2
  Product/1 -> Add/2
  Add/1 -> Product1/1
  R_2^T/1 -> Product1/2, Product2/2, Product3/1
  q - p_d/1 -> Product1/3
  Product1/1 -> Sum/1
  2/1 -> Sum/2
  p_d^s/1 -> Product2/3
  p_d^s^2/1 -> Product3/2
  Product3/1 -> Sum/3

== system NLPID/Guidance Systems/Path-following/Path/Ellipse path/p_d eq ==
  s : Inport
  r_x : Inport  Port=2
  r_y : Inport  Port=3
  origo_x : Inport  Port=4
  origo_y : Inport  Port=5
  k : Inport  Port=6
  Add : Sum  OutDataType=fixdt(1, 16)  OutScaling=2^-10
  Add1 : Sum  OutDataType=fixdt(1, 16)  OutScaling=2^-10
  Mux1 : Mux  Inputs=2
  Product : Product  OutDataType=fixdt(1, 16)  OutScaling=2^0  RndMeth=Zero
  Product1 : Product  OutDataType=fixdt(1, 16)  OutScaling=2^0  RndMeth=Zero
  Product2 : Product  OutDataType=fixdt(1, 16)  OutScaling=2^0  RndMeth=Zero
  cos(s) : Trigonometry  Operator=cos
  sin(s) : Trigonometry
  p_d : Outport
  wires:
  cos(s)/1 -> Product/2
  sin(s)/1 -> Product1/2
  Add/1 -> Mux1/1
  r_x/1 -> Product/1
  r_y/1 -> Product1/1
  Mux1/1 -> p_d/1
  origo_x/1 -> Add/2
  origo_y/1 -> Add1/2
  Product/1 -> Add/1
  Product1/1 -> Add1/1
  Add1/1 -> Mux1/2
  s/1 -> Product2/1
  k/1 -> Product2/2
  Product2/1 -> cos(s)/1, sin(s)/1

== system NLPID/Guidance Systems/Path-following/Path/Ellipse path/p_d^s eq ==
  s : Inport
  a : Inport  Port=2
  b : Inport  Port=3
  k : Inport  Port=4
  Gain : Gain  Gain=-1  ParameterDataType=fixdt(1, 16)  ParameterScaling=2^0  OutDataType=fixdt(1, 16)  OutScaling=2^0
  Mux1 : Mux  Inputs=2
  Product : Product  Inputs=3  OutDataType=fixdt(1, 16)  OutScaling=2^0  RndMeth=Zero
  Product1 : Product  Inputs=3  OutDataType=fixdt(1, 16)  OutScaling=2^0  RndMeth=Zero
  Product2 : Product  OutDataType=fixdt(1, 16)  OutScaling=2^0  RndMeth=Zero
  cos(s) : Trigonometry  Operator=cos
  sin(s) : Trigonometry
  p_d^s : Outport
  wires:
  s/1 -> Product2/1
  sin(s)/1 -> Product/2
  cos(s)/1 -> Product1/2
  Product/1 -> Gain/1
  Gain/1 -> Mux1/1
  Product1/1 -> Mux1/2
  a/1 -> Product/1
  b/1 -> Product1/1
  Mux1/1 -> p_d^s/1
  k/1 -> Product2/2, Product1/3, Product/3
  Product2/1 -> cos(s)/1, sin(s)/1

== system NLPID/Guidance Systems/Path-following/Path/Ellipse path/p_d^s^2 eq ==
  s : Inport
  a : Inport  Port=2
  b : Inport  Port=3
  k : Inport  Port=4
  Gain : Gain  Gain=-1  ParameterDataType=fixdt(1, 16)  ParameterScaling=2^0  OutDataType=fixdt(1, 16)  OutScaling=2^0
  Gain1 : Gain  Gain=-1  ParameterDataType=fixdt(1, 16)  ParameterScaling=2^0  OutDataType=fixdt(1, 16)  OutScaling=2^0
  Math Function : Math  Operator=square  OutDataType=fixdt(1, 16)  OutScaling=2^0  SaturateOnIntegerOverflow=on
  Mux2 : Mux  Inputs=2
  Product : Product  Inputs=3  OutDataType=fixdt(1, 16)  OutScaling=2^0  RndMeth=Zero
  Product1 : Product  Inputs=3  OutDataType=fixdt(1, 16)  OutScaling=2^0  RndMeth=Zero
  Product2 : Product  OutDataType=fixdt(1, 16)  OutScaling=2^0  RndMeth=Zero
  cos(s) : Trigonometry  Operator=cos
  sin(s) : Trigonometry
  p_d^s^2 : Outport
  wires:
  Product/1 -> Gain/1
  Gain/1 -> Mux2/1
  Product1/1 -> Gain1/1
  Gain1/1 -> Mux2/2
  cos(s)/1 -> Product/2
  sin(s)/1 -> Product1/2
  Mux2/1 -> p_d^s^2/1
  b/1 -> Product1/1
  a/1 -> Product/1
  k/1 -> Product2/2, Math Function/1
  s/1 -> Product2/1
  Product2/1 -> cos(s)/1, sin(s)/1
  Math Function/1 -> Product1/3, Product/3

== system NLPID/Guidance Systems/Path-following/Path/Ellipse path/p_d^s^3 eq ==
  s : Inport
  a : Inport  Port=2
  b : Inport  Port=3
  k : Inport  Port=4
  Constant : Constant  Value=3  OutDataType=fixdt(1, 16)  OutScaling=2^0
  Gain : Gain  Gain=-1  ParameterDataType=fixdt(1, 16)  ParameterScaling=2^0  OutDataType=fixdt(1, 16)  OutScaling=2^0
  Math Function : Math  Operator=pow  OutDataType=fixdt(1, 16)  OutScaling=2^0  SaturateOnIntegerOverflow=on
  Mux3 : Mux  Inputs=2
  Product : Product  Inputs=3  OutDataType=fixdt(1, 16)  OutScaling=2^0  RndMeth=Zero
  Product1 : Product  Inputs=3  OutDataType=fixdt(1, 16)  OutScaling=2^0  RndMeth=Zero
  Product2 : Product  OutDataType=fixdt(1, 16)  OutScaling=2^0  RndMeth=Zero
  cos(s)3 : Trigonometry  Operator=cos
  sin(s)3 : Trigonometry
  p_d^s^3 : Outport
  wires:
  Product1/1 -> Gain/1
  Gain/1 -> Mux3/2
  Mux3/1 -> p_d^s^3/1
  Product/1 -> Mux3/1
  cos(s)3/1 -> Product1/2
  sin(s)3/1 -> Product/2
  a/1 -> Product/1
  b/1 -> Product1/1
  k/1 -> Product2/2, Math Function/1
  s/1 -> Product2/1
  Product2/1 -> sin(s)3/1, cos(s)3/1
  Constant/1 -> Math Function/2
  Math Function/1 -> Product1/3, Product/3

== system NLPID/Guidance Systems/Path-following/Path/Ellipse path/|p_d^s| eq ==
  p_d^s : Inport
  Product : Product  Multiplication=Matrix(*)  OutDataType=fixdt(1, 16)  OutScaling=2^0  RndMeth=Zero
  Transpose : dspmtrx3/Transpose  SystemSampleTime=-1  Hermitian=off  overflowFlag=off
  sqrt : Math  Operator=sqrt  OutDataType=fixdt(1, 16)  OutScaling=2^0  SaturateOnIntegerOverflow=on
  |p_d^s| : Outport
  wires:
  Transpose/1 -> Product/1
  Product/1 -> sqrt/1
  sqrt/1 -> |p_d^s|/1
  p_d^s/1 -> Transpose/1, Product/2

== system NLPID/Guidance Systems/Path-following/Path/Path Switch workaround/p_d selcetor ==
  note: Path Selector == 1: Straight path
      | Path Selector == 0: Ellipse path
  Path Selector : Inport  OutDataType=fixdt(1, 16)  OutScaling=2^0
  p_d Straight path : Inport  Port=2  OutDataType=fixdt(1, 16)  OutScaling=2^0
  p_d Ellipse path : Inport  Port=3  OutDataType=fixdt(1, 16)  OutScaling=2^0
  1 - a : Sum  Inputs=+-  OutDataType=fixdt(1, 16)  OutScaling=2^-10
  Add : Sum  OutDataType=fixdt(1, 16)  OutScaling=2^-10
  Constant : Constant  OutDataType=fixdt(1, 16)  OutScaling=2^0
  p_d1 *a : Product  OutDataType=fixdt(1, 16)  OutScaling=2^0  RndMeth=Zero
  p_d2 * (1- a ) : Product  OutDataType=fixdt(1, 16)  OutScaling=2^0  RndMeth=Zero
  p_d : Outport
  wires:
  p_d2 * (1- a )/1 -> Add/2
  1 - a/1 -> p_d2 * (1- a )/2
  p_d1 *a/1 -> Add/1
  Constant/1 -> 1 - a/1
  Path Selector/1 -> 1 - a/2, p_d1 *a/2  "chosen path"
  Add/1 -> p_d/1
  p_d Straight path/1 -> p_d1 *a/1
  p_d Ellipse path/1 -> p_d2 * (1- a )/1

== system NLPID/Guidance Systems/Path-following/Path/Path Switch workaround/p_d^s selcetor ==
  note: Path Selector == 1: Straight path
      | Path Selector == 0: Ellipse path
  Path Selector : Inport  OutDataType=fixdt(1, 16)  OutScaling=2^0
  p_d^s Straight path : Inport  Port=2  OutDataType=fixdt(1, 16)  OutScaling=2^0
  p_d^s Ellipse path : Inport  Port=3  OutDataType=fixdt(1, 16)  OutScaling=2^0
  Add : Sum  OutDataType=fixdt(1, 16)  OutScaling=2^-10
  Constant : Constant  OutDataType=fixdt(1, 16)  OutScaling=2^0
  Product : Product  OutDataType=fixdt(1, 16)  OutScaling=2^0  RndMeth=Zero
  Product1 : Product  OutDataType=fixdt(1, 16)  OutScaling=2^0  RndMeth=Zero
  Subtract : Sum  Inputs=+-  OutDataType=fixdt(1, 16)  OutScaling=2^-10
  p_d^s : Outport
  wires:
  p_d^s Ellipse path/1 -> Product1/1
  p_d^s Straight path/1 -> Product/1
  Add/1 -> p_d^s/1
  Path Selector/1 -> Product/2, Subtract/2  "chosen path"
  Constant/1 -> Subtract/1
  Product/1 -> Add/1
  Subtract/1 -> Product1/2
  Product1/1 -> Add/2

== system NLPID/Guidance Systems/Path-following/Path/Path Switch workaround/p_d^s^3 selcetor ==
  note: Path Selector == 1: Straight path
      | Path Selector == 0: Ellipse path
  Path Selector : Inport  OutDataType=fixdt(1, 16)  OutScaling=2^0
  p_d^s^3 Straight path : Inport  Port=2  OutDataType=fixdt(1, 16)  OutScaling=2^0
  p_d^s^3 Ellipse path : Inport  Port=3  OutDataType=fixdt(1, 16)  OutScaling=2^0
  Add : Sum  OutDataType=fixdt(1, 16)  OutScaling=2^-10
  Constant : Constant  OutDataType=fixdt(1, 16)  OutScaling=2^0
  Product : Product  OutDataType=fixdt(1, 16)  OutScaling=2^0  RndMeth=Zero
  Product1 : Product  OutDataType=fixdt(1, 16)  OutScaling=2^0  RndMeth=Zero
  Subtract : Sum  Inputs=+-  OutDataType=fixdt(1, 16)  OutScaling=2^-10
  "p_d^s^3 " : Outport
  wires:
  p_d^s^3 Ellipse path/1 -> Product1/1
  p_d^s^3 Straight path/1 -> Product/1
  Add/1 -> "p_d^s^3 "/1
  Path Selector/1 -> Product/2, Subtract/2  "chosen path"
  Constant/1 -> Subtract/1
  Product/1 -> Add/1
  Subtract/1 -> Product1/2
  Product1/1 -> Add/2

== system NLPID/Guidance Systems/Path-following/Path/Path Switch workaround/p_ds^2 selcetor ==
  note: Path Selector == 1: Straight path
      | Path Selector == 0: Ellipse path
  Path Selector : Inport  OutDataType=fixdt(1, 16)  OutScaling=2^0
  p_ds^2  Straight path : Inport  Port=2  OutDataType=fixdt(1, 16)  OutScaling=2^0
  p_ds^2  Ellipse path : Inport  Port=3  OutDataType=fixdt(1, 16)  OutScaling=2^0
  Add : Sum  OutDataType=fixdt(1, 16)  OutScaling=2^-10
  Constant : Constant  OutDataType=fixdt(1, 16)  OutScaling=2^0
  Product : Product  OutDataType=fixdt(1, 16)  OutScaling=2^0  RndMeth=Zero
  Product1 : Product  OutDataType=fixdt(1, 16)  OutScaling=2^0  RndMeth=Zero
  Subtract : Sum  Inputs=+-  OutDataType=fixdt(1, 16)  OutScaling=2^-10
  "p_ds^2 " : Outport
  wires:
  p_ds^2  Ellipse path/1 -> Product1/1
  p_ds^2  Straight path/1 -> Product/1
  Add/1 -> "p_ds^2 "/1
  Path Selector/1 -> Product/2, Subtract/2  "chosen path"
  Constant/1 -> Subtract/1
  Product/1 -> Add/1
  Subtract/1 -> Product1/2
  Product1/1 -> Add/2

== system NLPID/Guidance Systems/Path-following/Path/Path Switch workaround/|p_d^s| selcetor ==
  note: Path Selector == 1: Straight path
      | Path Selector == 0: Ellipse path
  Path Selector : Inport  OutDataType=fixdt(1, 16)  OutScaling=2^0
  |p_d^s| Straight path : Inport  Port=2  OutDataType=fixdt(1, 16)  OutScaling=2^0
  |p_d^s| Ellipse path : Inport  Port=3  OutDataType=fixdt(1, 16)  OutScaling=2^0
  Add : Sum  OutDataType=fixdt(1, 16)  OutScaling=2^-10
  Constant : Constant  OutDataType=fixdt(1, 16)  OutScaling=2^0
  Product : Product  OutDataType=fixdt(1, 16)  OutScaling=2^0  RndMeth=Zero
  Product1 : Product  OutDataType=fixdt(1, 16)  OutScaling=2^0  RndMeth=Zero
  Subtract : Sum  Inputs=+-  OutDataType=fixdt(1, 16)  OutScaling=2^-10
  |p_d^s| : Outport
  wires:
  |p_d^s| Ellipse path/1 -> Product1/1
  |p_d^s| Straight path/1 -> Product/1
  Add/1 -> |p_d^s|/1
  Path Selector/1 -> Product/2, Subtract/2  "chosen path"
  Constant/1 -> Subtract/1
  Product/1 -> Add/1
  Subtract/1 -> Product1/2
  Product1/1 -> Add/2

== system NLPID/Guidance Systems/Path-following/Path/Straight path/p_d eq ==
  s : Inport
  x_1 : Inport  Port=2
  y_1 : Inport  Port=3
  x_2 : Inport  Port=4
  y_2 : Inport  Port=5
  (x_2 - x_1) * s : Product  OutDataType=fixdt(1, 16)  OutScaling=2^0  RndMeth=Zero
  (x_2 - x_1) * s + x_1 : Sum  OutDataType=fixdt(1, 16)  OutScaling=2^-10
  (y_2 - y_1) * s : Product  OutDataType=fixdt(1, 16)  OutScaling=2^0  RndMeth=Zero
  (y_2 - y_1) * s + y_1 : Sum  OutDataType=fixdt(1, 16)  OutScaling=2^-10
  Mux1 : Mux  Inputs=2
  x_2 - x_1 : Sum  Inputs=+-  OutDataType=fixdt(1, 16)  OutScaling=2^-10
  y_2 - y_1 : Sum  Inputs=+-  OutDataType=fixdt(1, 16)  OutScaling=2^-10
  p_d : Outport
  wires:
  (x_2 - x_1) * s + x_1/1 -> Mux1/1
  (y_2 - y_1) * s + y_1/1 -> Mux1/2
  (x_2 - x_1) * s/1 -> (x_2 - x_1) * s + x_1/1
  (y_2 - y_1) * s/1 -> (y_2 - y_1) * s + y_1/1
  x_2 - x_1/1 -> (x_2 - x_1) * s/1
  y_2 - y_1/1 -> (y_2 - y_1) * s/1
  s/1 -> (x_2 - x_1) * s/2, (y_2 - y_1) * s/2
  x_2/1 -> x_2 - x_1/1
  x_1/1 -> x_2 - x_1/2, (x_2 - x_1) * s + x_1/2
  y_2/1 -> y_2 - y_1/1
  y_1/1 -> y_2 - y_1/2, (y_2 - y_1) * s + y_1/2
  Mux1/1 -> p_d/1

== system NLPID/Guidance Systems/Path-following/Path/Straight path/p_d^s eq ==
  x_1 : Inport
  y_1 : Inport  Port=2
  x_2 : Inport  Port=3
  y_2 : Inport  Port=4
  Mux1 : Mux  Inputs=2
  x_2 - x_1 : Sum  Inputs=+-  OutDataType=fixdt(1, 16)  OutScaling=2^-10
  y_2 - y_1 : Sum  Inputs=+-  OutDataType=fixdt(1, 16)  OutScaling=2^-10
  p_d^s : Outport
  wires:
  Mux1/1 -> p_d^s/1
  x_2 - x_1/1 -> Mux1/1
  y_2 - y_1/1 -> Mux1/2
  x_2/1 -> x_2 - x_1/1
  x_1/1 -> x_2 - x_1/2
  y_2/1 -> y_2 - y_1/1
  y_1/1 -> y_2 - y_1/2

== system NLPID/Guidance Systems/Path-following/Path/Straight path/|p_d^s| eq ==
  p_d^s : Inport
  Product : Product  Multiplication=Matrix(*)  OutDataType=fixdt(1, 16)  OutScaling=2^0  RndMeth=Zero
  p_d^s^T : dspmtrx3/Transpose  SystemSampleTime=-1  Hermitian=off  overflowFlag=off
  sqrt : Math  Operator=sqrt  OutDataType=fixdt(1, 16)  OutScaling=2^0  SaturateOnIntegerOverflow=on
  |p_d^s| : Outport
  wires:
  p_d^s^T/1 -> Product/1
  Product/1 -> sqrt/1
  sqrt/1 -> |p_d^s|/1
  p_d^s/1 -> p_d^s^T/1, Product/2

== system NLPID/Guidance Systems/Path-following/Line-Of-Sight/LOS heading/psi_los eq/rad to pi2pi1 ==
  note: x
  note: r
  x (rad) : Inport  OutDataType=sfix(16)  OutScaling=2^0
  Constant : Constant  Value=2*180  OutDataType=sfix(16)  OutScaling=2^0
  Degrees to Radians : simulink_extras/Transformations/Degrees to Radians  SystemSampleTime=-1
  Gain : Gain  Gain=180  ParameterDataType=sfix(16)  ParameterScaling=2^0  OutDataType=sfix(16)  OutScaling=2^0  SaturateOnIntegerOverflow=on  OutDataTypeStr=Inherit: Same as input  ParamDataTypeStr=Inherit: Same as input
  Math Function : Math  Operator=rem  OutDataType=sfix(16)  OutScaling=2^0  SaturateOnIntegerOverflow=on
  Radians to Degrees : simulink_extras/Transformations/Radians to Degrees  SystemSampleTime=-1
  Saturation : Saturate  UpperLimit=1e10  LowerLimit=-1e10
  Sign : Signum
  Sum : Sum  Inputs=|+-  OutDataType=sfix(16)  OutScaling=2^0  SaturateOnIntegerOverflow=on
  Sum1 : Sum  Inputs=|++  OutDataType=sfix(16)  OutScaling=2^0  SaturateOnIntegerOverflow=on
  -pi to pi : Outport  OutDataType=sfix(16)  OutScaling=2^0
  wires:
  Saturation/1 -> Sum1/1, Sign/1
  x (rad)/1 -> Radians to Degrees/1
  Sign/1 -> Gain/1
  Gain/1 -> Sum/2, Sum1/2
  Sum1/1 -> Math Function/1
  Constant/1 -> Math Function/2
  Math Function/1 -> Sum/1
  Sum/1 -> Degrees to Radians/1
  Degrees to Radians/1 -> -pi to pi/1
  Radians to Degrees/1 -> Saturation/1

== system NLPID/Guidance Systems/Path-following/Line-Of-Sight/LOS heading/psi_los eq/rad to pi2pi2 ==
  note: x
  note: r
  x (rad) : Inport  OutDataType=sfix(16)  OutScaling=2^0
  Constant : Constant  Value=2*180  OutDataType=sfix(16)  OutScaling=2^0
  Degrees to Radians : simulink_extras/Transformations/Degrees to Radians  SystemSampleTime=-1
  Gain : Gain  Gain=180  ParameterDataType=sfix(16)  ParameterScaling=2^0  OutDataType=sfix(16)  OutScaling=2^0  SaturateOnIntegerOverflow=on  OutDataTypeStr=Inherit: Same as input  ParamDataTypeStr=Inherit: Same as input
  Math Function : Math  Operator=rem  OutDataType=sfix(16)  OutScaling=2^0  SaturateOnIntegerOverflow=on
  Radians to Degrees : simulink_extras/Transformations/Radians to Degrees  SystemSampleTime=-1
  Saturation : Saturate  UpperLimit=1e10  LowerLimit=-1e10
  Sign : Signum
  Sum : Sum  Inputs=|+-  OutDataType=sfix(16)  OutScaling=2^0  SaturateOnIntegerOverflow=on
  Sum1 : Sum  Inputs=|++  OutDataType=sfix(16)  OutScaling=2^0  SaturateOnIntegerOverflow=on
  -pi to pi : Outport  OutDataType=sfix(16)  OutScaling=2^0
  wires:
  Saturation/1 -> Sum1/1, Sign/1
  x (rad)/1 -> Radians to Degrees/1
  Sign/1 -> Gain/1
  Gain/1 -> Sum/2, Sum1/2
  Sum1/1 -> Math Function/1
  Constant/1 -> Math Function/2
  Math Function/1 -> Sum/1
  Sum/1 -> Degrees to Radians/1
  Degrees to Radians/1 -> -pi to pi/1
  Radians to Degrees/1 -> Saturation/1

== system NLPID/Guidance Systems/Path-following/Line-Of-Sight/LOS heading/psi_los eq/rad to pi2pi3 ==
  note: r
  note: x
  x (rad) : Inport  OutDataType=sfix(16)  OutScaling=2^0
  Constant : Constant  Value=2*180  OutDataType=sfix(16)  OutScaling=2^0
  Degrees to Radians : simulink_extras/Transformations/Degrees to Radians  SystemSampleTime=-1
  Gain : Gain  Gain=180  ParameterDataType=sfix(16)  ParameterScaling=2^0  OutDataType=sfix(16)  OutScaling=2^0  SaturateOnIntegerOverflow=on  OutDataTypeStr=Inherit: Same as input  ParamDataTypeStr=Inherit: Same as input
  Math Function : Math  Operator=rem  OutDataType=sfix(16)  OutScaling=2^0  SaturateOnIntegerOverflow=on
  Radians to Degrees : simulink_extras/Transformations/Radians to Degrees  SystemSampleTime=-1
  Saturation : Saturate  UpperLimit=1e10  LowerLimit=-1e10
  Sign : Signum
  Sum : Sum  Inputs=|+-  OutDataType=sfix(16)  OutScaling=2^0  SaturateOnIntegerOverflow=on
  Sum1 : Sum  Inputs=|++  OutDataType=sfix(16)  OutScaling=2^0  SaturateOnIntegerOverflow=on
  -pi to pi : Outport  OutDataType=sfix(16)  OutScaling=2^0
  wires:
  Radians to Degrees/1 -> Saturation/1
  Degrees to Radians/1 -> -pi to pi/1
  Sum/1 -> Degrees to Radians/1
  Math Function/1 -> Sum/1
  Constant/1 -> Math Function/2
  Sum1/1 -> Math Function/1
  Gain/1 -> Sum1/2, Sum/2
  Sign/1 -> Gain/1
  x (rad)/1 -> Radians to Degrees/1
  Saturation/1 -> Sign/1, Sum1/1
